simulink model "projector"  (R2020a)
settings: Solver=ode15s  StartTime=0.0  StopTime=200  RelTol=1e-3  AbsTol=1e-3
libraries: fl_lib x12, nesl_utility x5
settings Model: Creator=Afraz  LastModifiedBy=Afraz
settings SolverCC: AutoScaleAbsTol=off
settings DebuggingCC: SymbolicDimsDataTypeCodeGenerationDiagnostic=none
settings SFSimCC: CustomCodeUndefinedFunction=UseInterfaceOnly
settings SimscapeCC: SimscapeLogType=all  SimscapeLogSimulationStatistics=on  SimscapeLogDataHistory=10000

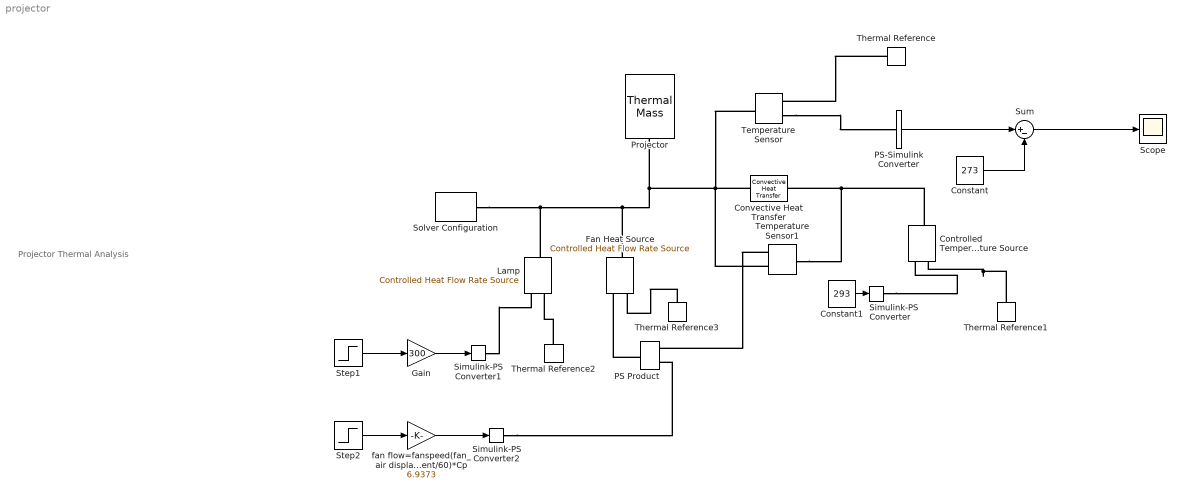
== system projector ==
  note: Projector Thermal Analysis
  Constant : Constant  Value=273
  Constant1 : Constant  Value=293
  Controlled Temperature Source : fl_lib/Thermal/Thermal Sources/Controlled Temperature Source
  Convective Heat Transfer : fl_lib/Thermal/Thermal Elements/Convective Heat Transfer  area=1.5e-02 m^2  heat_tr_coeff=200 W/(m^2 * K)  T_specify=off  T_priority=None  T=0 K  T_nominal_specify=off  T_nominal_unit=K  T_nominal_value=1  Q_specify=off  Q_priority=None  Q=0 W  Q_nominal_specify=off  Q_nominal_unit=W  Q_nominal_value=1
  Fan Heat Source : fl_lib/Thermal/Thermal Sources/Controlled Heat Flow Rate Source
  Gain : Gain  Gain=300
  Lamp : fl_lib/Thermal/Thermal Sources/Controlled Heat Flow Rate Source
  PS Product : fl_lib/Physical Signals/Functions/PS Product
  PS-Simulink Converter : nesl_utility/PS-Simulink Converter  PhysicalDomain=network_engine_domain  SubClassName=ps_output  LeftPortType=input  RightPortType=output  PseudoPeriodic=off  Frequencies=[]  Unit=K  AffineConversion=off
      settings: SourceProductBaseCode=MT,SS
  Projector : fl_lib/Thermal/Thermal Elements/Thermal Mass  mass=.05 kg  sp_heat=1005.4 J/kg/K  T_specify=on  T_priority=High  T=273 K  T_nominal_specify=off  T_nominal_unit=K  T_nominal_value=1  Q_specify=on  Q_priority=None  Q=0 W  Q_nominal_specify=off  Q_nominal_unit=W  Q_nominal_value=1
  Scope : Scope
  Simulink-PS Converter : nesl_utility/Simulink-PS Converter  PhysicalDomain=network_engine_domain  SubClassName=ps_input  LeftPortType=input  RightPortType=output  PseudoPeriodic=off  Frequencies=[]  NoiseDistribution=none  NoiseParameters=[]  Unit=K  AffineConversion=off  FilteringAndDerivatives=provide  SimscapeFilterOrder=1  InputFilterTimeConstant=0.001  UdotUserProvided=0
      settings: SourceProductBaseCode=MT,SS
  Simulink-PS Converter1 : nesl_utility/Simulink-PS Converter  PhysicalDomain=network_engine_domain  SubClassName=ps_input  LeftPortType=input  RightPortType=output  PseudoPeriodic=off  Frequencies=[]  NoiseDistribution=none  NoiseParameters=[]  Unit=W  AffineConversion=off  FilteringAndDerivatives=provide  SimscapeFilterOrder=1  InputFilterTimeConstant=0.001  UdotUserProvided=0
      settings: SourceProductBaseCode=MT,SS
  Simulink-PS Converter2 : nesl_utility/Simulink-PS Converter  PhysicalDomain=network_engine_domain  SubClassName=ps_input  LeftPortType=input  RightPortType=output  PseudoPeriodic=off  Frequencies=[]  NoiseDistribution=none  NoiseParameters=[]  Unit=W/K  AffineConversion=off  FilteringAndDerivatives=provide  SimscapeFilterOrder=1  InputFilterTimeConstant=0.001  UdotUserProvided=0
      settings: SourceProductBaseCode=MT,SS
  Solver Configuration : nesl_utility/Solver Configuration  PhysicalDomain=network_engine_domain  SubClassName=solver  LeftPortType=input  RightPortType=generic  Tones=[]  Harmonics=[]  SimulateNoise=off  Profile=off  UseLocalSampling=off  EnableSwitchedLinearOptims=on  FrequencyDomain=off  UseCCode=off  RelTol=0.001  AbsTol=1e-06  MinStep=1e-09  ToWorkspace=off  RevertToSquareIcSolve=off  NumHomotopyIterations=100  PhasorMode=off  PhasorModeNumHarmonics=1  DoDC=off  ResidualTolerance=1e-09  UseLocalSolver=off  LocalSolverChoice=NE_BACKWARD_EULER_ADVANCER  LocalSolverSampleTime=0.001  DoFixedCost=off  MaxNonlinIter=3  MaxModeIter=2  LinearAlgebra=auto  EquationFormulation=NE_TIME_EF  DelaysMemoryBudget=1024  AutomaticFiltering=on  FilteringTimeConstant=0.001  PartitionStorageMethod=AS_NEEDED  PartitionMemoryBudget=1024  PartitionMethod=ROBUST
      settings: SourceProductBaseCode=MT,SS
  Step1 : Step  Time=60  SampleTime=0
  Step2 : Step  Time=160  SampleTime=0
  Sum : Sum  Inputs=|+-
  Temperature Sensor : fl_lib/Thermal/Thermal Sensors/Temperature Sensor
  Temperature Sensor1 : fl_lib/Thermal/Thermal Sensors/Temperature Sensor
  Thermal Reference{,1..3} (4 alike) : fl_lib/Thermal/Thermal Elements/Thermal Reference
  fan flow=fanspeed(fan_air displacement/60)*Cp : Gain  Gain=6.9373
  wires:
  Constant/1 -> Sum/2
  PS-Simulink Converter/1 -> Sum/1
  Sum/1 -> Scope/1
  Constant1/1 -> Simulink-PS Converter/1
  Step1/1 -> Gain/1
  Gain/1 -> Simulink-PS Converter1/1
  fan flow=fanspeed(fan_air displacement/60)*Cp/1 -> Simulink-PS Converter2/1
  Step2/1 -> fan flow=fanspeed(fan_air displacement/60)*Cp/1
  connections:
  Convective Heat Transfer/LConn1 -- Temperature Sensor1/RConn1 -- Temperature Sensor/LConn1 -- Fan Heat Source/LConn1 -- Lamp/LConn1 -- Solver Configuration/RConn1 -- Projector/LConn1
  Controlled Temperature Source/LConn1 -- Temperature Sensor1/LConn1 -- Convective Heat Transfer/RConn1
  Thermal Reference/LConn1 -- Temperature Sensor/RConn1
  Temperature Sensor/RConn2 -- PS-Simulink Converter/LConn1
  Thermal Reference1/LConn1 -- Controlled Temperature Source/RConn2
  Simulink-PS Converter/RConn1 -- Controlled Temperature Source/RConn1
  Thermal Reference2/LConn1 -- Lamp/RConn2
  Simulink-PS Converter1/RConn1 -- Lamp/RConn1
  Temperature Sensor1/RConn2 -- PS Product/LConn2
  Simulink-PS Converter2/RConn1 -- PS Product/LConn1
  PS Product/RConn1 -- Fan Heat Source/RConn1
  Thermal Reference3/LConn1 -- Fan Heat Source/RConn2
